simulink model "evaluateParamVar"  (R2016b)
settings: Solver=VariableStepAuto  StartTime=0.0  StopTime=0.4  RelTol=1e-3
values from neighbouring files (symbols this model uses):
  plant = tf(1,[0.01 1])    [transferfunDisObserver_sim.m]
  plantWithVar = plant*1/1.5    [transferfunDisObserver_sim.m]
settings Model: Creator=Yu  LastModifiedBy=Yu

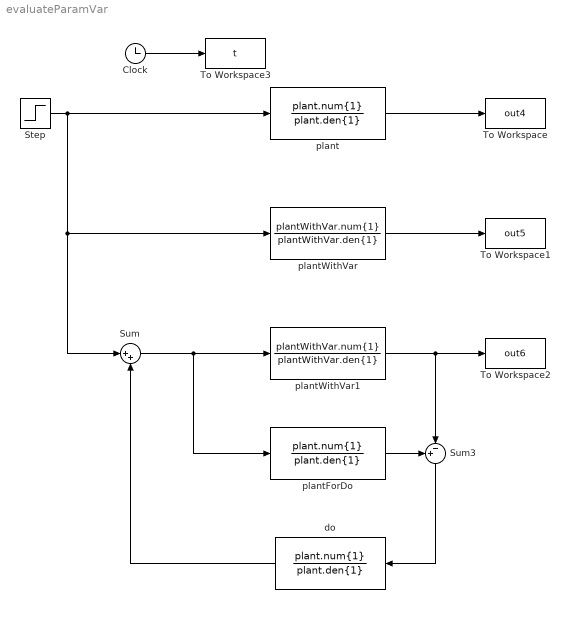
== system evaluateParamVar ==
  Clock : Clock
  Step : Step  Time=0.01  SampleTime=0
  Sum : Sum  Inputs=|++
  Sum3 : Sum  Inputs=+-|
  To Workspace : ToWorkspace  VariableName=out4  SampleTime=-1
  To Workspace1 : ToWorkspace  VariableName=out5  SampleTime=-1
  To Workspace2 : ToWorkspace  VariableName=out6  SampleTime=-1
  To Workspace3 : ToWorkspace  VariableName=t  SampleTime=-1
  do : TransferFcn  Numerator=plant.num{1}  Denominator=plant.den{1}
  plant : TransferFcn  Numerator=plant.num{1}  Denominator=plant.den{1}
  plantForDo : TransferFcn  Numerator=plant.num{1}  Denominator=plant.den{1}
  plantWithVar : TransferFcn  Numerator=plantWithVar.num{1}  Denominator=plantWithVar.den{1}
  plantWithVar1 : TransferFcn  Numerator=plantWithVar.num{1}  Denominator=plantWithVar.den{1}
  wires:
  Step/1 -> plant/1, Sum/1, plantWithVar/1
  Sum/1 -> plantForDo/1, plantWithVar1/1
  do/1 -> Sum/2
  plantWithVar1/1 -> Sum3/2, To Workspace2/1
  plant/1 -> To Workspace/1
  plantWithVar/1 -> To Workspace1/1
  plantForDo/1 -> Sum3/1
  Sum3/1 -> do/1
  Clock/1 -> To Workspace3/1
